simulink library "brakes"  (R2025b)
settings: Solver=VariableStepAuto  StartTime=0.0  StopTime=10.0  RelTol=1e-3
settings Model: Creator=jessi  LastModifiedBy=jessi

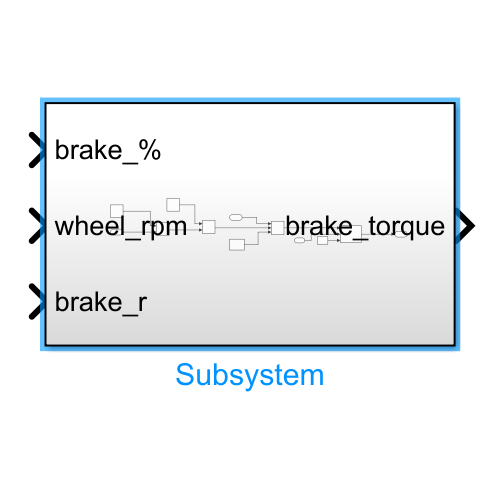
[thumbnail: Simulink's stored preview of the top-level diagram]
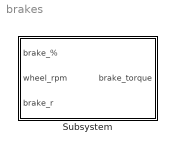
== system brakes ==
  Subsystem : Subsystem

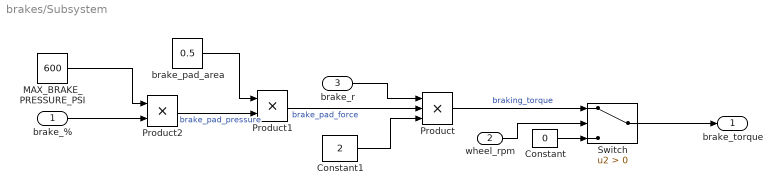
== system brakes/Subsystem ==
  brake_% : Inport  Unit=%  PortDimensions=1
  wheel_rpm : Inport  Port=2  Unit=rpm  PortDimensions=4
  brake_r : Inport  Port=3  Unit=m  PortDimensions=1
  Constant : Constant  Value=0
  Constant1 : Constant  Value=2
  MAX_BRAKE_PRESSURE_PSI : Constant  Value=600
  Product : Product  Inputs=3
  Product1 : Product
  Product2 : Product
  Switch : Switch  Criteria=u2 > Threshold  SaturateOnIntegerOverflow=off  InputSameDT=off
  brake_pad_area : Constant  Value=0.5
  brake_torque : Outport
  wires:
  MAX_BRAKE_PRESSURE_PSI/1 -> Product2/1
  brake_%/1 -> Product2/2
  Product2/1 -> Product1/2  "brake_pad_pressure"
  wheel_rpm/1 -> Switch/2
  Constant/1 -> Switch/3
  Switch/1 -> brake_torque/1
  brake_pad_area/1 -> Product1/1
  Product1/1 -> Product/2  "brake_pad_force"
  brake_r/1 -> Product/1
  Product/1 -> Switch/1  "braking_torque"
  Constant1/1 -> Product/3
